simulink model "attitudePropagate"  (R2023b)
settings: Solver=VariableStepAuto  StartTime=0.0  StopTime=Tfinal  RelTol=1e-3
model workspace (MAT data in the model file):
  attitdueType = "euler"
  attitudeType = "euler"
  sequence = "313"
  u0 = [2.91319105247; 0.437912021527; 0.275895246399]
settings Model: Creator=stanforduser  LastModifiedBy=annahylbert

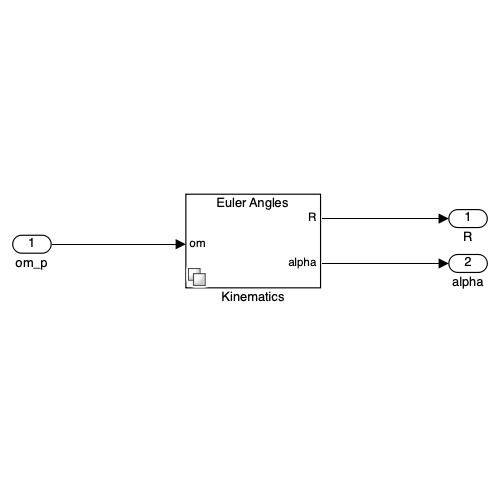
[thumbnail: Simulink's stored preview of the top-level diagram]
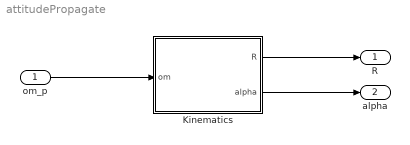
== system attitudePropagate ==
  om_p : Inport
  Kinematics : Subsystem  Variant=on
  R : Outport
  alpha : Outport  Port=2
  wires:
  om_p/1 -> Kinematics/1(om)
  Kinematics/1(R) -> R/1
  Kinematics/2(alpha) -> alpha/1

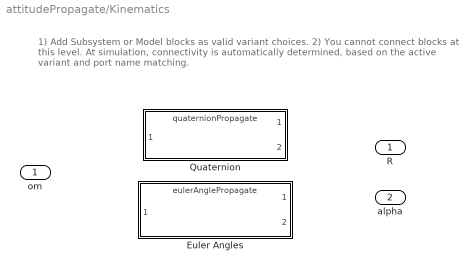
== system attitudePropagate/Kinematics ==
  note: 1) Add Subsystem or Model blocks as valid variant choices.
      | 2) You cannot connect blocks at this level. At simulation, connectivity is automatically
      | determined, based on the active variant and port name matching.
  om : Inport
  Euler Angles : ModelReference  ModelNameDialog=eulerAnglePropagate.slx  SimulationMode=Normal  VariantControl="attitudeType==\"euler\""  ModelReferenceVersion=1.139
  Quaternion : ModelReference  ModelNameDialog=quaternionPropagate.slx  SimulationMode=Normal  VariantControl="attitudeType==\"quat\""  ModelReferenceVersion=1.22
  R : Outport
  alpha : Outport  Port=2
